simulink model "helikopter_maketa"  (Simulink 8.6)
settings: Solver=ode45  StartTime=0.0  StopTime=70  RelTol=1e-3
values from neighbouring files (symbols this model uses):
  bh = 0.05    [helikopter_maketa_paraametri.m]    (also in helikopter_maketa_parametri.m)
  bv = 0.05    [helikopter_maketa_paraametri.m]    (also in helikopter_maketa_parametri.m)
  dz1_z = 0.07    [helikopter_maketa_paraametri.m]    (also in helikopter_maketa_parametri.m)
  dz2_z = 0.08    [helikopter_maketa_paraametri.m]    (also in helikopter_maketa_parametri.m)
  g = 9.81    [helikopter_maketa_paraametri.m]    (also in helikopter_maketa_parametri.m)
  I = m1*l1^2 + m2*l2^2 + m3*l3^2    (= 0.0128174)    [helikopter_maketa_paraametri.m]    (also in helikopter_maketa_parametri.m)
  K1_u = 0.14/l1    (= 0.474576271186)    [helikopter_maketa_paraametri.m]    (also in helikopter_maketa_parametri.m)
  K1_z = 0.014*l1/l2    (= 0.01475)    [helikopter_maketa_paraametri.m]    (also in helikopter_maketa_parametri.m)
  K2_z = 0.05    [helikopter_maketa_paraametri.m]    (also in helikopter_maketa_parametri.m)
  l1 = 0.295    [helikopter_maketa_paraametri.m]    (also in helikopter_maketa_parametri.m)
  l2 = 0.280    (= 0.28)    [helikopter_maketa_paraametri.m]    (also in helikopter_maketa_parametri.m)
  l3 = 0.120    (= 0.12)    [helikopter_maketa_paraametri.m]    (also in helikopter_maketa_parametri.m)
  m1 = 0.120    (= 0.12)    [helikopter_maketa_paraametri.m]    (also in helikopter_maketa_parametri.m)
  m2 = 0.020    (= 0.02)    [helikopter_maketa_paraametri.m]    (also in helikopter_maketa_parametri.m)
  m3 = 0.056    [helikopter_maketa_paraametri.m]    (also in helikopter_maketa_parametri.m)
  theta0 = -5*pi/180    (= -0.0872664625997)    [helikopter_maketa_paraametri.m]    (also in helikopter_maketa_parametri.m = -0.872664625997)
  theta_max = 50*pi/180    (= 0.872664625997)    [helikopter_maketa_paraametri.m]    (also in helikopter_maketa_parametri.m)
  theta_min = -50*pi/180    (= -0.872664625997)    [helikopter_maketa_paraametri.m]    (also in helikopter_maketa_parametri.m)
  u1_max = 12    [helikopter_maketa_paraametri.m]    (also in helikopter_maketa_parametri.m)
  u1_min = 0    [helikopter_maketa_paraametri.m]    (also in helikopter_maketa_parametri.m)
  u2_max = 5    [helikopter_maketa_paraametri.m]    (also in helikopter_maketa_parametri.m)
  u2_min = -5    [helikopter_maketa_paraametri.m]    (also in helikopter_maketa_parametri.m)
settings Model: Creator=damjan  LastModifiedBy=Branko
settings DebuggingCC: SolverPrmCheckMsg=none  FcnCallInpInsideContextMsg=EnableAllAsWarning

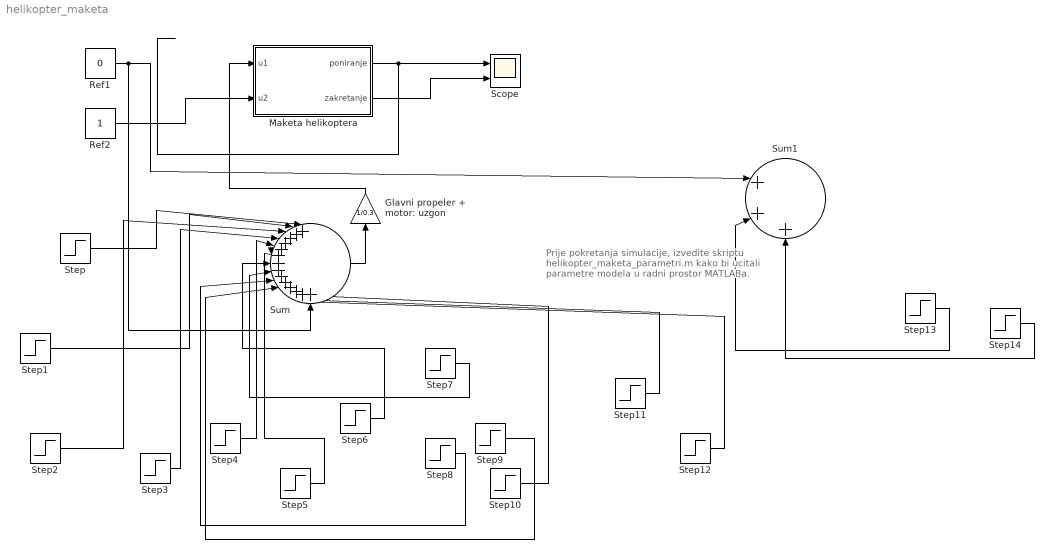
== system helikopter_maketa ==
  note: Prije pokretanja simulacije, izvedite skriptu
      | helikopter_maketa_parametri.m kako bi
      | ucitali parametre modela u radni prostor
      | MATLABa.
  Glavni propeler + motor: uzgon : Gain  Gain=1/0.3
  Maketa helikoptera : Subsystem
  Ref1 : Constant  Value=0
  Ref2 : Constant
  Scope : Scope  NumInputPorts=2
  Step : Step  After=0.3  SampleTime=0
  Step1 : Step  Time=6  After=0.3  SampleTime=0
  Step10 : Step  Time=51  After=0.3  SampleTime=0
  Step11 : Step  Time=56  After=0.3  SampleTime=0
  Step12 : Step  Time=61  After=0.3  SampleTime=0
  Step13 : Step  Time=12  SampleTime=0
  Step14 : Step  Time=24  After=-1  SampleTime=0
  Step2 : Step  Time=11  After=0.3  SampleTime=0
  Step3 : Step  Time=16  After=0.3  SampleTime=0
  Step4 : Step  Time=21  After=0.3  SampleTime=0
  Step5 : Step  Time=26  After=0.3  SampleTime=0
  Step6 : Step  Time=31  After=0.3  SampleTime=0
  Step7 : Step  Time=36  After=0.3  SampleTime=0
  Step8 : Step  Time=41  After=0.3  SampleTime=0
  Step9 : Step  Time=46  After=0.3  SampleTime=0
  Sum : Sum  Inputs=|++++++++++++++
  Sum1 : Sum  Inputs=|+++
  wires:
  Maketa helikoptera/1(poniranje) -> Scope/1
  Maketa helikoptera/2(zakretanje) -> Scope/2
  Ref2/1 -> Maketa helikoptera/2(u2)
  Step/1 -> Sum/1
  Step1/1 -> Sum/2
  Step2/1 -> Sum/3
  Step3/1 -> Sum/4
  Step4/1 -> Sum/5
  Step5/1 -> Sum/6
  Step6/1 -> Sum/7
  Step7/1 -> Sum/8
  Step8/1 -> Sum/9
  Step9/1 -> Sum/10
  Step10/1 -> Sum/11
  Step11/1 -> Sum/12
  Step12/1 -> Sum/13
  Step13/1 -> Sum1/2
  Step14/1 -> Sum1/3
  Ref1/1 -> Sum/14, Sum1/1
  Sum/1 -> Glavni propeler + motor: uzgon/1
  Glavni propeler + motor: uzgon/1 -> Maketa helikoptera/1(u1)

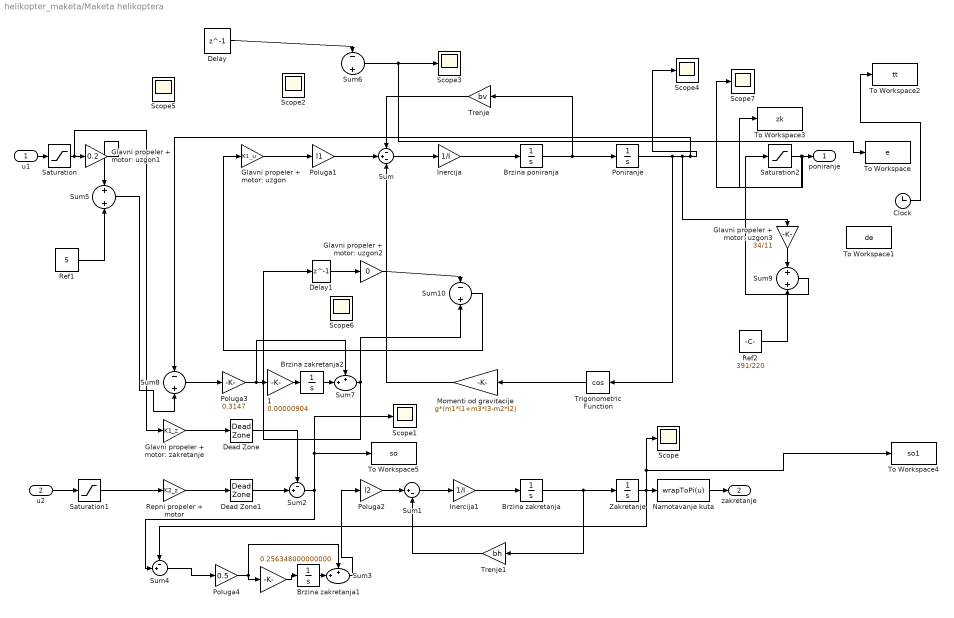
== system helikopter_maketa/Maketa helikoptera ==
  u1 : Inport
  u2 : Inport  Port=2
  " " : Gain  Gain=0.256348000000000
  " 1" : Gain  Gain=0.00000904
  Brzina poniranja : Integrator
  Brzina zakretanja : Integrator
  Brzina zakretanja1 : Integrator
  Brzina zakretanja2 : Integrator
  Clock : Clock
  Dead Zone : DeadZone  LowerValue=-dz1_z  UpperValue=dz1_z  SaturateOnIntegerOverflow=on
  Dead Zone1 : DeadZone  LowerValue=-dz2_z  UpperValue=dz2_z  SaturateOnIntegerOverflow=on
  Delay : Delay  DelayLength=1  InitialCondition=0  SampleTime=0.001
  Delay1 : Delay  DelayLength=1  InitialCondition=0  SampleTime=0.001
  Glavni propeler + motor: uzgon : Gain  Gain=K1_u
  Glavni propeler + motor: uzgon1 : Gain  Gain=0.2
  Glavni propeler + motor: uzgon2 : Gain  Gain=0
  Glavni propeler + motor: uzgon3 : Gain  Gain=34/11
  Glavni propeler + motor: zakretanje : Gain  Gain=K1_z
  Inercija : Gain  Gain=1/I
  Inercija1 : Gain  Gain=1/I
  Momenti od gravitacije : Gain  Gain=g*(m1*l1+m3*l3-m2*l2)
  Namotavanje kuta : MATLABFcn  MATLABFcn=wrapToPi(u)
  Poluga1 : Gain  Gain=l1
  Poluga2 : Gain  Gain=l2
  Poluga3 : Gain  Gain=0.3147
  Poluga4 : Gain  Gain=0.5
  Poniranje : Integrator  InitialCondition=theta0  LimitOutput=on  UpperSaturationLimit=theta_max  LowerSaturationLimit=theta_min  ContinuousStateAttributes='theta'
  Ref1 : Constant  Value=5
  Ref2 : Constant  Value=391/220
  Repni propeler + motor : Gain  Gain=K2_z
  Saturation : Saturate  UpperLimit=u1_max  LowerLimit=u1_min
  Saturation1 : Saturate  UpperLimit=u2_max  LowerLimit=u2_min
  Saturation2 : Saturate  UpperLimit=0.8727  LowerLimit=-0.8727
  Scope{,1..7} (8 alike) : Scope
  Sum : Sum  Inputs=-+-
  Sum1 : Sum  Inputs=|+-
  Sum10 : Sum  Inputs=-+
  Sum2 : Sum  Inputs=-+|
  Sum3 : Sum  Inputs=++|
  Sum4 : Sum  Inputs=-+|
  Sum5 : Sum
  Sum6 : Sum  Inputs=-+
  Sum7 : Sum  Inputs=++|
  Sum8 : Sum  Inputs=-+
  Sum9 : Sum
  To Workspace : ToWorkspace  VariableName=e  SampleTime=-1
      settings: Save2DSignal=2-D array (concatenate along first dimension)
  To Workspace1 : ToWorkspace  VariableName=de  SampleTime=-1
      settings: Save2DSignal=2-D array (concatenate along first dimension)
  To Workspace2 : ToWorkspace  VariableName=tt  SampleTime=-1
      settings: Save2DSignal=2-D array (concatenate along first dimension)
  To Workspace3 : ToWorkspace  VariableName=zk  SampleTime=-1
      settings: Save2DSignal=2-D array (concatenate along first dimension)
  To Workspace4 : ToWorkspace  VariableName=so1  SampleTime=-1
      settings: Save2DSignal=2-D array (concatenate along first dimension)
  To Workspace5 : ToWorkspace  VariableName=so  SampleTime=-1
      settings: Save2DSignal=2-D array (concatenate along first dimension)
  Trenje : Gain  Gain=bv
  Trenje1 : Gain  Gain=bh
  Trigonometric Function : Trigonometry  Operator=cos
  Zakretanje : Integrator  ContinuousStateAttributes='phi'
  poniranje : Outport
  zakretanje : Outport  Port=2
  wires:
  Inercija/1 -> Brzina poniranja/1
  Brzina poniranja/1 -> Poniranje/1, Trenje/1
  Trenje/1 -> Sum/1
  Sum/1 -> Inercija/1
  Trigonometric Function/1 -> Momenti od gravitacije/1
  Momenti od gravitacije/1 -> Sum/3
  Glavni propeler + motor: uzgon/1 -> Poluga1/1
  Glavni propeler + motor: zakretanje/1 -> Dead Zone/1
  Sum1/1 -> Inercija1/1
  Inercija1/1 -> Brzina zakretanja/1
  Brzina zakretanja/1 -> Zakretanje/1, Trenje1/1
  Trenje1/1 -> Sum1/2
  Repni propeler + motor/1 -> Dead Zone1/1
  Dead Zone1/1 -> Sum2/2
  Dead Zone/1 -> Sum2/1
  Poluga2/1 -> Sum1/1
  u2/1 -> Saturation1/1
  u1/1 -> Saturation/1
  Saturation1/1 -> Repni propeler + motor/1
  Namotavanje kuta/1 -> zakretanje/1
  Poluga4/1 -> Sum3/1, " "/1
  " "/1 -> Brzina zakretanja1/1
  Brzina zakretanja1/1 -> Sum3/2
  Sum3/1 -> Poluga2/1
  Sum4/1 -> Poluga4/1
  Sum2/1 -> To Workspace5/1, Scope1/1, Sum4/2
  Zakretanje/1 -> To Workspace4/1, Scope/1, Sum4/1, Namotavanje kuta/1
  Poluga1/1 -> Sum/2
  Sum6/1 -> To Workspace/1, Scope3/1
  Delay/1 -> Sum6/1
  Clock/1 -> To Workspace2/1
  Poniranje/1 -> Trigonometric Function/1, Glavni propeler + motor: uzgon3/1, Sum8/1, Scope4/1
  Poluga3/1 -> Sum7/1, " 1"/1
  " 1"/1 -> Brzina zakretanja2/1
  Brzina zakretanja2/1 -> Sum7/2
  Sum8/1 -> Poluga3/1
  Sum5/1 -> Sum8/2
  Ref1/1 -> Sum5/2
  Saturation/1 -> Glavni propeler + motor: zakretanje/1, Glavni propeler + motor: uzgon1/1
  Glavni propeler + motor: uzgon1/1 -> Sum5/1
  Ref2/1 -> Sum9/2
  Sum10/1 -> Glavni propeler + motor: uzgon/1
  Delay1/1 -> Glavni propeler + motor: uzgon2/1
  Sum7/1 -> Sum10/2, Delay1/1
  Glavni propeler + motor: uzgon2/1 -> Sum10/1
  Sum9/1 -> Saturation2/1
  Glavni propeler + motor: uzgon3/1 -> Sum9/1
  Saturation2/1 -> Scope7/1, To Workspace3/1, poniranje/1
